simulink model "sampleModel1742"  (R2023a)
settings: Solver=VariableStepAuto  StartTime=0.0  StopTime=10.0  RelTol=1e-3
libraries: hdlsllib x7, simulink x3
settings Model: Creator=user1  LastModifiedBy=user1

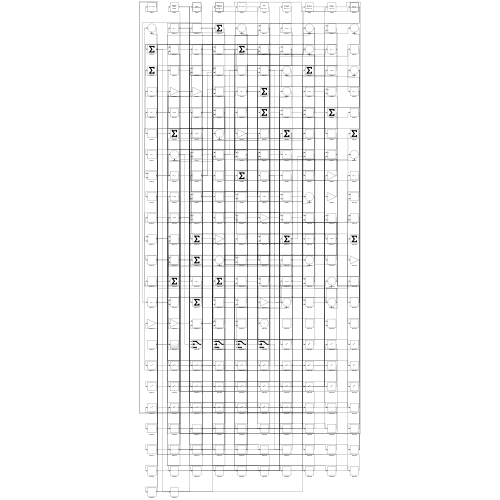
[thumbnail: Simulink's stored preview of the top-level diagram]
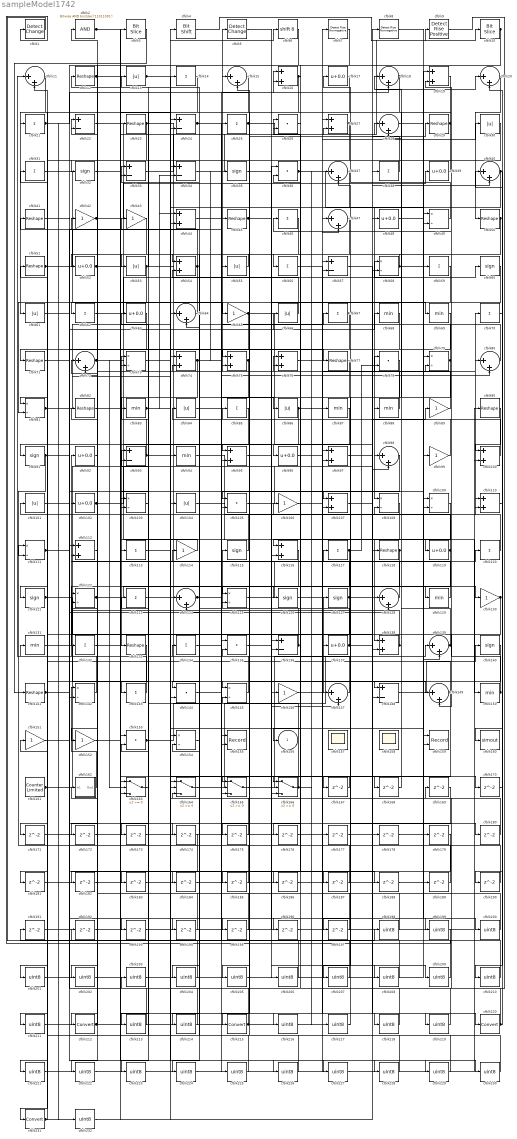
== system sampleModel1742 ==
  cfblk1 : simulink/Logic and Bit Operations/Detect Change  vinit=0  OutDataTypeStr=boolean
      settings: LibrarySourceBlock=|
      | hdlsllib/Logic and Bit
      | Operations/Detect
      | Change
  cfblk10 : hdlsllib/Logic and Bit Operations/Bit Slice  lidx=7  ridx=0
  cfblk{16,19,27,44,54,74..76,95,97,100,107,110,112,116,138} (16 alike) : Sum
  cfblk{13,30,53,55,61,66,84,86,101,104} (10 alike) : Abs  SaturateOnIntegerOverflow=off
  cfblk{17,39,48,52,63,92,96,102,119,137} (10 alike) : Bias  Bias=0.0  SaturateOnIntegerOverflow=off
  cfblk{49,58,73,79,81,103,108..109,111,122,125,142,145,154} (14 alike) : Product  Inputs=*/  RndMeth=Zero  SaturateOnIntegerOverflow=on
  cfblk{26,36,78,105,135,144,153} (7 alike) : DotProduct  OutDataTypeStr=Inherit: Inherit via internal rule
  cfblk{42..43,65,89,99,106,114,130,146,151..152} (11 alike) : Gain
  cfblk{11,15,18,20,28,37,40,47,64,72,80,98,124,128,139,147,149} (17 alike) : Sum  Inputs=|++
  cfblk{14,21,25,31,38,46,56,59,62,67,70,85,113,117,120,123,132,134,143} (19 alike) : Sum  Inputs=+
  cfblk{32,35,60,91,115,121,126..127,140} (9 alike) : Signum
  cfblk{12,23,29,41,45,50..51,71,77,82,90,118,133,141} (14 alike) : Reshape
  cfblk{68..69,83,87..88,94,129,131,150} (9 alike) : MinMax
  cfblk{22,24,33..34,57,93,136,148} (8 alike) : Sum  Inputs=+-
  cfblk155 : Record  FileSettingsInternal="{\"entries\":[{\"content\":{\"excelSettings\":{\"content\":{},\"type\":\"Streamout.ExcelSettings\"}},\"type\":\"Streamout.FileSettingStorage\",\"uuid\":\"\"}],\"packageUris\":[\"http:\\/\\/schema.mathworks.com\\/mf0\\/streamout_blocks\\/R2020a\"],\"version\":\"1.0\"}"  Layout=[1 1]  SignalsInternal="{\"entries\":[{\"content\":{\"signals\":[{\"content\":{\"blockPath\":[],\"dimensions\":[1],\"domain\":\"\",\"lineColor\":\"#a2142f\",\"plots\":[1],\"port\":1,\"signalID\":3560,\"signalName\":\"XY Graph:1\"},\"type\":\"RecordBlkView.Signal\",\"uuid\":\"\"},{\"content\":{\"blockPath\":[],\"dimensions\":[1],\"domain\":\"\",\"lineColor\":\"#139fff\",\"plots\":[1],\"port\":2,\"signalID\":3563,\"signalName\":\"XY Graph:2\"},\"type\":\"RecordBlkView.Signal\",\"uuid\":\"\"}]},\"type\":\"RecordBlkView.InputSignals\",\"uuid\":\"\"}],\"packageUris\":[\"http:\\/\\/schema.mathworks.com\\/mf0\\/streamout_blocks\\/R2020a\"],\"version\":\"1.0\"}"  VisualizationBindings="{\"xyplotplugin\":{\"info\":[{\"series\":[{\"bindingParametersList\":[{\"parameter\":\"X-Axis\",\"signalID\":3560,\"signalName\":\"XY Graph:1\"},{\"parameter\":\"Y-Axis\",\"signalID\":3563,\"signalName\":\"XY Graph:2\"}],\"seriesID\":33812}],\"subplotID\":1}]}}"  CompatibilityTag=XY  st=-1
  cfblk157 : Scope
      settings: Floating=on
  cfblk158 : Scope
      settings: Floating=on
  cfblk159 : Record  FileSettingsInternal="{\"entries\":[{\"content\":{\"excelSettings\":{\"content\":{},\"type\":\"Streamout.ExcelSettings\"}},\"type\":\"Streamout.FileSettingStorage\",\"uuid\":\"\"}],\"packageUris\":[\"http:\\/\\/schema.mathworks.com\\/mf0\\/streamout_blocks\\/R2020a\"],\"version\":\"1.0\"}"  Layout=[1 1]  SignalsInternal="{\"entries\":[{\"content\":{\"signals\":[{\"content\":{\"blockPath\":[],\"dimensions\":[1],\"domain\":\"\",\"lineColor\":\"#a2142f\",\"plots\":[1],\"port\":1,\"signalID\":3568,\"signalName\":\"XY Graph:1\"},\"type\":\"RecordBlkView.Signal\",\"uuid\":\"\"},{\"content\":{\"blockPath\":[],\"dimensions\":[1],\"domain\":\"\",\"lineColor\":\"#139fff\",\"plots\":[1],\"port\":2,\"signalID\":3571,\"signalName\":\"XY Graph:2\"},\"type\":\"RecordBlkView.Signal\",\"uuid\":\"\"}]},\"type\":\"RecordBlkView.InputSignals\",\"uuid\":\"\"}],\"packageUris\":[\"http:\\/\\/schema.mathworks.com\\/mf0\\/streamout_blocks\\/R2020a\"],\"version\":\"1.0\"}"  VisualizationBindings="{\"xyplotplugin\":{\"info\":[{\"series\":[{\"bindingParametersList\":[{\"parameter\":\"X-Axis\",\"signalID\":3568,\"signalName\":\"XY Graph:1\"},{\"parameter\":\"Y-Axis\",\"signalID\":3571,\"signalName\":\"XY Graph:2\"}],\"seriesID\":25713}],\"subplotID\":1}]}}"  CompatibilityTag=XY  st=-1
  cfblk160 : ToWorkspace  VariableName=simout  SaveFormat=Timeseries  SampleTime=-1
  cfblk161 : hdlsllib/Sources/Counter Limited  uplimit=7  tsamp=-1
  cfblk162 : Subsystem
      settings: LibrarySourceBlock=|
      | hdlsllib/Ports &
      | Subsystems/Subsystem
  cfblk{163..166} (4 alike) : Switch  SaturateOnIntegerOverflow=off  InputSameDT=off
  cfblk{167..197} (31 alike) : Delay  SampleTime=1
  cfblk{198..211,213..214,216..219,221..230,232} (31 alike) : DataTypeConversion  OutDataTypeStr=uint8  SaturateOnIntegerOverflow=off  RndMeth=Floor
  cfblk2 : simulink/Logic and Bit Operations/Bitwise Operator  logicop=AND  UseBitMask=on  BitMask=bin2dec('11011001')  BitMaskRealWorld=Stored Integer
      settings: LibrarySourceBlock=|
      | hdlsllib/Logic and Bit
      | Operations/Bitwise
      | Operator
  cfblk{212,215,220,231} (4 alike) : DataTypeConversion  SaturateOnIntegerOverflow=off  RndMeth=Floor
  cfblk3 : hdlsllib/Logic and Bit Operations/Bit Slice  lidx=7  ridx=0
  cfblk4 : hdlsllib/Logic and Bit Operations/Bit Shift  mode=Shift Left Logical  N=0
  cfblk5 : simulink/Logic and Bit Operations/Detect Change  vinit=0  OutDataTypeStr=boolean
      settings: LibrarySourceBlock=|
      | hdlsllib/Logic and Bit
      | Operations/Detect
      | Change
  cfblk6 : ArithShift  BitShiftNumber=8
  cfblk7 : hdlsllib/Logic and Bit Operations/Detect Rise Nonnegative  vinit=0  OutDataTypeStr=boolean
  cfblk8 : hdlsllib/Logic and Bit Operations/Detect Rise Nonnegative  vinit=0  OutDataTypeStr=boolean
  cfblk9 : hdlsllib/Logic and Bit Operations/Detect Rise Positive  vinit=0  OutDataTypeStr=boolean
  cfblk156 : Outport  VectorParamsAs1DForOutWhenUnconnected=off
  wires:
  cfblk11/1 -> cfblk61/1
  cfblk23/1 -> cfblk145/1, cfblk211/1
  cfblk67/1 -> cfblk163/3, cfblk172/1
  cfblk40/1 -> cfblk108/1, cfblk160/1, cfblk44/2
  cfblk122/1 -> cfblk129/1, cfblk16/2
  cfblk74/1 -> cfblk133/1, cfblk67/1, cfblk35/1
  cfblk18/1 -> cfblk143/1, cfblk181/1
  cfblk104/1 -> cfblk70/1
  cfblk49/1 -> cfblk17/1
  cfblk115/1 -> cfblk31/1
  cfblk57/1 -> cfblk220/1
  cfblk142/1 -> cfblk11/1
  cfblk22/1 -> cfblk119/1
  cfblk164/1 -> cfblk139/1
  cfblk131/1 -> cfblk148/1
  cfblk93/1 -> cfblk94/1, cfblk73/1, cfblk159/2
  cfblk136/1 -> cfblk115/1, cfblk12/1
  cfblk12/1 -> cfblk219/1, cfblk226/1
  cfblk163/1 -> cfblk93/1
  cfblk88/1 -> cfblk5/1
  cfblk150/1 -> cfblk46/1, cfblk76/1, cfblk101/1
  cfblk10/1 -> cfblk96/1, cfblk186/1
  cfblk37/1 -> cfblk215/1
  cfblk64/1 -> cfblk62/1
  cfblk143/1 -> cfblk92/1
  cfblk130/1 -> cfblk149/2, cfblk201/1
  cfblk99/1 -> cfblk84/1
  cfblk31/1 -> cfblk104/1
  cfblk145/1 -> cfblk114/1
  cfblk108/1 -> cfblk138/1
  cfblk42/1 -> cfblk39/1, cfblk165/2
  cfblk50/1 -> cfblk98/1, cfblk166/3
  cfblk4/1 -> cfblk9/1
  cfblk27/1 -> cfblk125/1, cfblk75/2
  cfblk161/1 -> cfblk38/1, cfblk66/1
  cfblk86/1 -> cfblk91/1, cfblk156/1, cfblk147/1, cfblk30/1
  cfblk39/1 -> cfblk32/1
  cfblk21/1 -> cfblk71/1, cfblk18/2, cfblk232/1
  cfblk96/1 -> cfblk27/1
  cfblk149/1 -> cfblk51/1, cfblk18/1, cfblk175/1
  cfblk63/1 -> cfblk121/1
  cfblk117/1 -> cfblk144/1, cfblk78/2
  cfblk3/1 -> cfblk141/1
  cfblk29/1 -> cfblk21/1, cfblk95/1
  cfblk102/1 -> cfblk47/1, cfblk195/1
  cfblk114/1 -> cfblk113/1
  cfblk51/1 -> cfblk45/1, cfblk73/2
  cfblk81/1 -> cfblk6/1, cfblk4/1
  cfblk80/1 -> cfblk36/2
  cfblk33/1 -> cfblk20/1
  cfblk141/1 -> cfblk128/2, cfblk174/1
  cfblk112/1 -> cfblk212/1
  cfblk58/1 -> cfblk59/1, cfblk52/1
  cfblk121/1 -> cfblk120/1, cfblk148/2
  cfblk52/1 -> cfblk136/1, cfblk22/1
  cfblk20/1 -> cfblk50/1
  cfblk107/1 -> cfblk29/1
  cfblk116/1 -> cfblk136/2
  cfblk105/1 -> cfblk89/1
  cfblk166/1 -> cfblk83/1, cfblk177/1
  cfblk153/1 -> cfblk55/1, cfblk68/1
  cfblk61/1 -> cfblk77/1
  cfblk35/1 -> cfblk107/1
  cfblk65/1 -> cfblk118/1, cfblk165/3
  cfblk91/1 -> cfblk111/2, cfblk193/1
  cfblk14/1 -> cfblk231/1
  cfblk82/1 -> cfblk3/1
  cfblk90/1 -> cfblk100/1
  cfblk83/1 -> cfblk107/2, cfblk34/2, cfblk44/1
  cfblk111/1 -> cfblk43/1, cfblk188/1
  cfblk69/1 -> cfblk116/1
  cfblk128/1 -> cfblk26/1
  cfblk146/1 -> cfblk127/1
  cfblk152/1 -> cfblk25/1
  cfblk43/1 -> cfblk53/1
  cfblk25/1 -> cfblk27/2, cfblk69/1
  cfblk139/1 -> cfblk78/1, cfblk19/2
  cfblk125/1 -> cfblk47/2
  cfblk26/1 -> cfblk56/1
  cfblk54/1 -> cfblk13/1, cfblk81/2, cfblk93/2
  cfblk129/1 -> cfblk72/1
  cfblk19/1 -> cfblk88/1
  cfblk2/1 -> cfblk24/2, cfblk194/1
  cfblk73/1 -> cfblk144/2
  cfblk95/1 -> cfblk60/1
  cfblk162/1(Out1) -> cfblk142/1
  cfblk94/1 -> cfblk150/1
  cfblk165/1 -> cfblk80/1
  cfblk15/1 -> cfblk103/1
  cfblk53/1 -> cfblk125/2, cfblk28/1, cfblk152/1, cfblk33/2
  cfblk62/1 -> cfblk49/2
  cfblk13/1 -> cfblk109/2, cfblk170/1
  cfblk126/1 -> cfblk79/2
  cfblk137/1 -> cfblk40/2, cfblk33/1
  cfblk120/1 -> cfblk110/1
  cfblk147/1 -> cfblk63/1
  cfblk34/1 -> cfblk10/1
  cfblk84/1 -> cfblk155/1
  cfblk109/1 -> cfblk126/1
  cfblk76/1 -> cfblk130/1
  cfblk45/1 -> cfblk146/1, cfblk147/2
  cfblk24/1 -> cfblk80/2, cfblk86/1
  cfblk72/1 -> cfblk164/1, cfblk163/2
  cfblk154/1 -> cfblk64/2
  cfblk17/1 -> cfblk65/1
  cfblk46/1 -> cfblk105/1
  cfblk38/1 -> cfblk15/2
  cfblk100/1 -> cfblk74/2
  cfblk132/1 -> cfblk117/1
  cfblk75/1 -> cfblk95/2, cfblk185/1
  cfblk148/1 -> cfblk140/1
  cfblk119/1 -> cfblk42/1, cfblk76/2, cfblk124/2, cfblk197/1
  cfblk36/1 -> cfblk159/1, cfblk217/1
  cfblk48/1 -> cfblk99/1
  cfblk98/1 -> cfblk165/1
  cfblk124/1 -> cfblk16/1, cfblk187/1
  cfblk44/1 -> cfblk155/2
  cfblk30/1 -> cfblk75/1
  cfblk16/1 -> cfblk166/1, cfblk81/1
  cfblk68/1 -> cfblk103/2
  cfblk79/1 -> cfblk41/1, cfblk224/1
  cfblk55/1 -> cfblk54/1
  cfblk66/1 -> cfblk54/2
  cfblk41/1 -> cfblk105/2
  cfblk118/1 -> cfblk132/1, cfblk58/1
  cfblk127/1 -> cfblk85/1, cfblk166/2, cfblk110/2
  cfblk6/1 -> cfblk142/2
  cfblk56/1 -> cfblk149/1
  cfblk89/1 -> cfblk2/1
  cfblk138/1 -> cfblk122/1, cfblk28/2
  cfblk78/1 -> cfblk167/1
  cfblk167/1 -> cfblk164/2
  cfblk113/1 -> cfblk168/1
  cfblk168/1 -> cfblk108/2
  cfblk170/1 -> cfblk40/1
  cfblk133/1 -> cfblk171/1
  cfblk171/1 -> cfblk79/1
  cfblk172/1 -> cfblk64/1
  cfblk103/1 -> cfblk173/1
  cfblk175/1 -> cfblk74/1
  cfblk77/1 -> cfblk176/1
  cfblk176/1 -> cfblk26/2
  cfblk177/1 -> cfblk128/1
  cfblk178/1 -> cfblk109/1
  cfblk71/1 -> cfblk180/1
  cfblk180/1 -> cfblk24/1
  cfblk181/1 -> cfblk36/1
  cfblk92/1 -> cfblk182/1
  cfblk182/1 -> cfblk49/1
  cfblk60/1 -> cfblk183/1
  cfblk47/1 -> cfblk184/1
  cfblk185/1 -> cfblk154/2
  cfblk186/1 -> cfblk19/1
  cfblk187/1 -> cfblk122/2
  cfblk188/1 -> cfblk139/2
  cfblk28/1 -> cfblk189/1
  cfblk189/1 -> cfblk111/1
  cfblk70/1 -> cfblk190/1
  cfblk190/1 -> cfblk164/3
  cfblk191/1 -> cfblk100/2
  cfblk192/1 -> cfblk116/2
  cfblk193/1 -> cfblk58/2
  cfblk194/1 -> cfblk72/2
  cfblk195/1 -> cfblk163/1
  cfblk32/1 -> cfblk196/1
  cfblk196/1 -> cfblk138/2
  cfblk197/1 -> cfblk22/2
  cfblk1/1 -> cfblk198/1
  cfblk198/1 -> cfblk137/1
  cfblk173/1 -> cfblk199/1
  cfblk199/1 -> cfblk1/1
  cfblk8/1 -> cfblk200/1
  cfblk200/1 -> cfblk102/1
  cfblk201/1 -> cfblk8/1
  cfblk7/1 -> cfblk202/1
  cfblk202/1 -> cfblk48/1
  cfblk9/1 -> cfblk203/1
  cfblk203/1 -> cfblk7/1
  cfblk179/1 -> cfblk204/1
  cfblk204/1 -> cfblk153/1
  cfblk140/1 -> cfblk205/1
  cfblk205/1 -> cfblk179/1
  cfblk135/1 -> cfblk206/1
  cfblk206/1 -> cfblk154/1
  cfblk169/1 -> cfblk207/1
  cfblk207/1 -> cfblk135/1
  cfblk5/1 -> cfblk208/1
  cfblk208/1 -> cfblk135/2
  cfblk97/1 -> cfblk209/1
  cfblk209/1 -> cfblk11/2
  cfblk110/1 -> cfblk210/1
  cfblk210/1 -> cfblk97/1
  cfblk211/1 -> cfblk97/2
  cfblk212/1 -> cfblk34/1, cfblk124/1, cfblk162/1(In1)
  cfblk183/1 -> cfblk213/1
  cfblk213/1 -> cfblk112/1
  cfblk85/1 -> cfblk214/1
  cfblk214/1 -> cfblk112/2
  cfblk215/1 -> cfblk82/1, cfblk15/1
  cfblk184/1 -> cfblk216/1
  cfblk216/1 -> cfblk37/1
  cfblk217/1 -> cfblk37/2
  cfblk106/1 -> cfblk218/1
  cfblk218/1 -> cfblk192/1
  cfblk219/1 -> cfblk106/1
  cfblk220/1 -> cfblk169/1, cfblk20/2, cfblk153/2
  cfblk59/1 -> cfblk221/1
  cfblk221/1 -> cfblk57/1
  cfblk174/1 -> cfblk222/1
  cfblk222/1 -> cfblk57/2
  cfblk87/1 -> cfblk223/1
  cfblk223/1 -> cfblk90/1
  cfblk224/1 -> cfblk87/1
  cfblk134/1 -> cfblk225/1
  cfblk225/1 -> cfblk191/1
  cfblk226/1 -> cfblk134/1
  cfblk123/1 -> cfblk227/1
  cfblk227/1 -> cfblk98/2
  cfblk101/1 -> cfblk228/1
  cfblk228/1 -> cfblk123/1
  cfblk151/1 -> cfblk229/1
  cfblk229/1 -> cfblk145/2
  cfblk144/1 -> cfblk230/1
  cfblk230/1 -> cfblk151/1
  cfblk231/1 -> cfblk178/1, cfblk131/1, cfblk23/1
  cfblk232/1 -> cfblk14/1

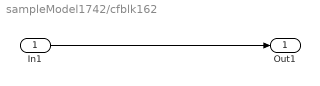
== system sampleModel1742/cfblk162 ==
  In1 : Inport
  Out1 : Outport
  wires:
  In1/1 -> Out1/1
